simulink model "PDFedbackControl"  (R2017a)
settings: Solver=ode45  StartTime=0.0  StopTime=5  MaxStep=0.001  RelTol=1e-3
values from neighbouring files (symbols this model uses):
  K1 = 6.5    [fric.mat]    (also in lab5Script.m; parmEstimate2ndOrderTF.m = y1/(1-MCal(zetaEst,wnEst,t1)); projection.m = ySample(1)/(1-MCal(zetaEst,wnEst,tSample(1))))
  K2 = 6    [fric.mat]    (also in lab5Script.m; parmEstimate2ndOrderTF.m = y2/(1-MCal(zetaEst,wnEst,t2)); projection.m = ySample(2)/(1-MCal(zetaEst,wnEst,tSample(2))))
  Kamp = 2.4    [lab5Script.m]
  Kpot = 1.6    [lab5Script.m]
  Ktach = 0.03    [lab5Script.m]
settings Model: Creator=maherna4  LastModifiedBy=maherna4

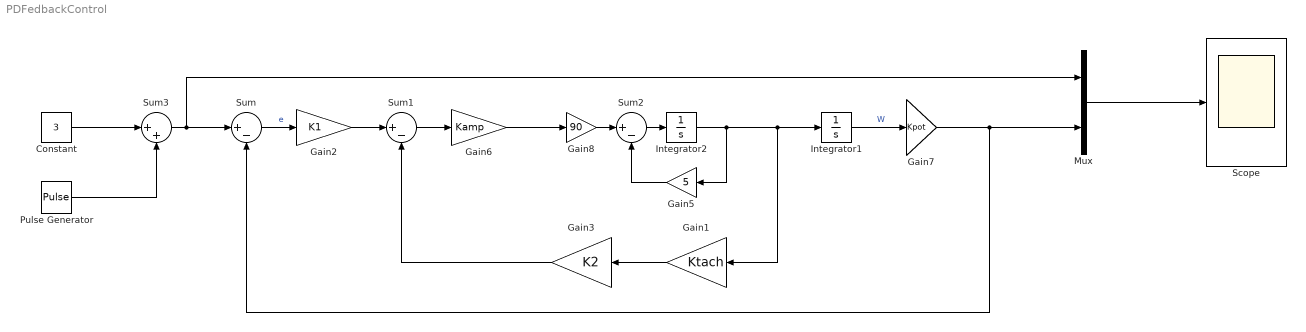
== system PDFedbackControl ==
  Constant : Constant  Value=3
  Gain1 : Gain  Gain=Ktach
  Gain2 : Gain  Gain=K1
  Gain3 : Gain  Gain=K2
  Gain5 : Gain  Gain=5
  Gain6 : Gain  Gain=Kamp
  Gain7 : Gain  Gain=Kpot
  Gain8 : Gain  Gain=90
  Integrator1 : Integrator
  Integrator2 : Integrator
  Mux : Mux  Inputs=2
  Pulse Generator : DiscretePulseGenerator  PulseType=Time based  Amplitude=2  PulseWidth=50
  Scope : Scope
  Sum : Sum  Inputs=|+-
  Sum1 : Sum  Inputs=|+-
  Sum2 : Sum  Inputs=|+-
  Sum3 : Sum  Inputs=|++
  wires:
  Gain3/1 -> Sum1/2
  Sum/1 -> Gain2/1  "e"
  Integrator1/1 -> Gain7/1  "W"
  Gain7/1 -> Sum/2, Mux/2
  Gain1/1 -> Gain3/1
  Sum1/1 -> Gain6/1
  Sum2/1 -> Integrator2/1
  Integrator2/1 -> Gain1/1, Integrator1/1, Gain5/1
  Gain5/1 -> Sum2/2
  Gain8/1 -> Sum2/1
  Gain6/1 -> Gain8/1
  Mux/1 -> Scope/1
  Constant/1 -> Sum3/1
  Pulse Generator/1 -> Sum3/2
  Sum3/1 -> Mux/1, Sum/1
  Gain2/1 -> Sum1/1
